simulink model "small_differential_catamaran"  (R2024a)
settings: Solver=VariableStepAuto  StartTime=0.0  StopTime=10.0  RelTol=1e-3
undefined symbols (not defined in the file or in its folder): ss_x, ss_yaw
settings Model: Creator=luka  LastModifiedBy=luka

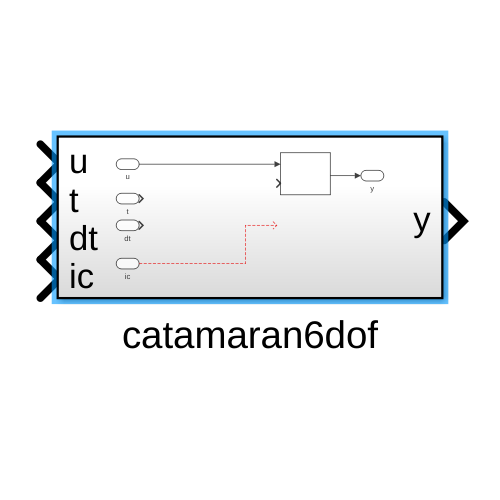
[thumbnail: Simulink's stored preview of the top-level diagram]
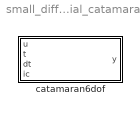
== system small_differential_catamaran ==
  catamaran6dof : Subsystem

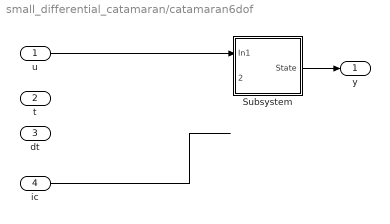
== system small_differential_catamaran/catamaran6dof ==
  u : Inport  PortDimensions=2
  t : Inport  Port=2
  dt : Inport  Port=3
  ic : Inport  Port=4
  Subsystem : Subsystem
  y : Outport  PortDimensions=6
  wires:
  ic/1 -> ?
  Subsystem/1(State) -> y/1
  u/1 -> Subsystem/1(In1)

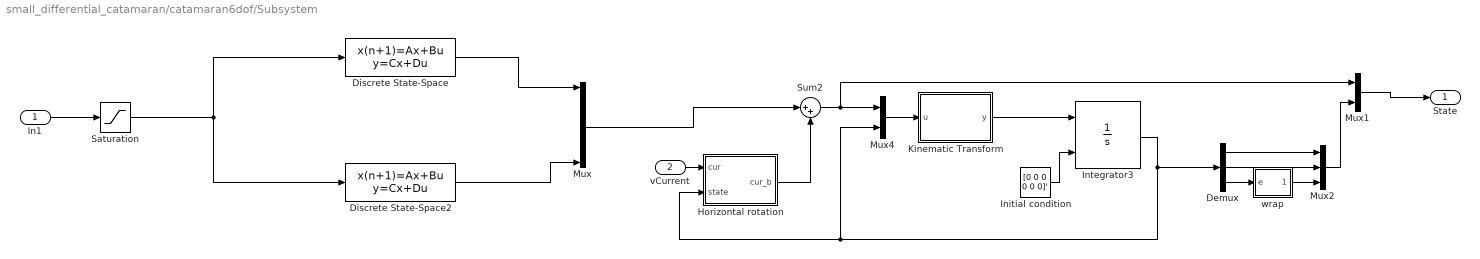
== system small_differential_catamaran/catamaran6dof/Subsystem ==
  In1 : Inport
  vCurrent : Inport  Port=2
  Demux : Demux  Outputs=3
  Discrete State-Space : DiscreteStateSpace  A=ss_x.A  B=ss_x.B  C=ss_x.C  D=ss_x.D  SampleTime=ss_x.Ts
  Discrete State-Space2 : DiscreteStateSpace  A=ss_yaw.A  B=ss_yaw.B  C=ss_yaw.C  D=ss_yaw.D  SampleTime=ss_yaw.Ts
  Horizontal rotation : MATLAB Function  TreatAsAtomicUnit=on
  Initial condition : Constant  Value=[0 0 0 0 0 0]'
  Integrator3 : Integrator  InitialConditionSource=external
  Kinematic Transform : MATLAB Function  TreatAsAtomicUnit=on
  Mux : Mux  Inputs=6
  Mux1 : Mux  Inputs=2
  Mux2 : Mux  Inputs=3
  Mux4 : Mux  Inputs=2
  Saturation : Saturate  UpperLimit=1  LowerLimit=-1
  Sum2 : Sum  Inputs=|++
  wrap : MATLAB Function  TreatAsAtomicUnit=on
  State : Outport
  wires:
  Saturation/1 -> Discrete State-Space/1, Discrete State-Space2/1
  Mux2/1 -> Mux1/2
  Demux/2 -> Mux2/2
  Demux/1 -> Mux2/1
  wrap/1(ew) -> Mux2/3
  Demux/3 -> wrap/1(e)
  Discrete State-Space/1 -> Mux/1
  Mux1/1 -> State/1
  Horizontal rotation/1(cur_b) -> Sum2/2
  Mux/1 -> Sum2/1
  Integrator3/1 -> Mux4/2, Horizontal rotation/2(state), Demux/1
  Mux4/1 -> Kinematic Transform/1(u)
  vCurrent/1 -> Horizontal rotation/1(cur)
  Sum2/1 -> Mux4/1, Mux1/1
  Initial condition/1 -> Integrator3/2
  Kinematic Transform/1(y) -> Integrator3/1
  Discrete State-Space2/1 -> Mux/6
  In1/1 -> Saturation/1

== matlab function small_differential_catamaran/catamaran6dof/Subsystem/Kinematic Transform ==
  data: u input; y output
function y = fcn(u)
%#codegen
if (length(u)<12) 
    y = zeros(12,1);
    return;
end

input = u;
% Read inputs
u = input(1,1);
v = input(2,1);
w = input(3,1);
p = input(4,1);
q = input(5,1);
r = input(6,1);

%x = input(7,1);
%y = input(8,1);
%z = input(9,1);
phi = input(10,1);
theta = input(11,1);
Psi = input(12,1);

DOF6 = 1; % Select degrees of freedom

tmp1 = []; tmp2 = [];

if DOF6 == 1
    
    % Rotation matrix
    R_x_phi = [1 0 0; 0 cos(phi) sin(phi); 0 -sin(phi) cos(phi)];
    R_y_theta = [cos(theta) 0 -sin(theta); 0 1 0; sin(theta) 0 cos(theta)];% Provjeri matrice
    R_z_psi = [cos(Psi) sin(Psi) 0; -sin(Psi) cos(Psi) 0; 0 0 1];
    
    % Linear velocity transform
    J1 = R_z_psi.'*R_y_theta.'*R_x_phi.';
    
    % Angular velocity transform    
    tmp1 = R_x_phi(:,2);
    tmp1 = [0 0 0; tmp1.'; 0 0 0].';
    
    tmp2 = R_x_phi*R_y_theta;
    tmp2 = tmp2(:,3);
    tmp2 = [0 0 0; 0 0 0; tmp2.'].';
    
    J2 = inv(diag([1 0 0])+tmp1+tmp2);
    
elseif DOF6 == 0
    
    % Rotation matrix
    R_x_phi = eye(3);
    R_y_theta = eye(3);
    R_z_psi = [cos(Psi) sin(Psi) 0; -sin(Psi) cos(Psi) 0; 0 0 1]; % Provjeri matrice
    
    % Linear velocity transform
    J1 = R_z_psi.'*R_y_theta.'*R_x_phi.';
    
    % Angular velocity transform 
    tmp1 = R_x_phi(:,2);
    tmp1 = [0 0 0; tmp1.'; 0 0 0].';
    
    tmp2 = R_x_phi*R_y_theta;
    tmp2 = tmp2(:,3);
    tmp2 = [0 0 0; 0 0 0; tmp2.'].';
    
    J2 = inv(diag([1 0 0])+tmp1+tmp2);
    
end

eta1 = J1*[u v w].';
eta2 = J2*[p q r].';


y = [eta1.' eta2.'].';

== matlab function small_differential_catamaran/catamaran6dof/Subsystem/wrap ==
  data: e input; ew output
function ew = wrap(e)

ew = mod(e, 2*pi);

if ew > pi
   ew = -2*pi + ew;
elseif ew <= -pi 
   ew = 2*pi + ew;
end

== matlab function small_differential_catamaran/catamaran6dof/Subsystem/Horizontal rotation ==
  data: cur input; cur_b output; state input
function cur_b = fcn(cur, state)
cur_b = zeros(6,1);
Psi = state(6,1);
R_z_psi = [cos(Psi) sin(Psi); -sin(Psi) cos(Psi)];

cur_ne_b = R_z_psi*cur;
cur_b(1) = cur_ne_b(1);
cur_b(2) = cur_ne_b(2);
